simulink model "aerial_controller"  (R2026a)
settings: Solver=ode4  StopTime=2000  FixedStep=0.005
InitFcn:
  | addpath('C:\Users\banda\Documents\MATLAB\UAUV Control\Aerial');run('C:\Users\banda\Documents\MATLAB\UAUV Control\Aerial\aerial_init.m');run('C:\Users\banda\Documents\MATLAB\UAUV Control\Aerial\trajectory_aerial.m');update_trajectory_size('aerial_controller', size(trajectory,1));
values from neighbouring files (symbols this model uses):
  A_face = [0.1; 0.1; 0.2]    [aerial_init.m]    (also in underwater_init.m = [W_box * H_box)
  att_lim = 0.45    [aerial_init.m]
  Cd = [1.28; 1.28; 1.28]    [aerial_init.m]    (also in underwater_init.m = [1.2; 1.2; 1.5])
  g = 9.81    [aerial_init.m]    (also in underwater_init.m)
  i_lim_phi = 10.0    (= 10)    [aerial_init.m]
  i_lim_psi = 5.0    (= 5)    [aerial_init.m]
  i_lim_r = 5.0    (= 5)    [aerial_init.m]
  i_lim_t = 5.0    (= 5)    [aerial_init.m]
  i_lim_theta = 10.0    (= 10)    [aerial_init.m]
  i_lim_z = 10.0    (= 10)    [aerial_init.m]
  I_matrix = diag([Ixx, Iyy, Izz])    [aerial_init.m]
  Jr = 6.0e-5    (= 6e-05)    [aerial_init.m]
  Kd_phi = 18.39    [aerial_init.m]
  Kd_psi = 20.71    [aerial_init.m]
  Kd_r = 1.0    (= 1)    [aerial_init.m]
  Kd_t = 1.1    [aerial_init.m]
  Kd_theta = 45.6    [aerial_init.m]
  Kd_z = 2.0    (= 2)    [aerial_init.m]
  Ki_phi = 0.3    [aerial_init.m]
  Ki_psi = 0.1    [aerial_init.m]
  Ki_r = 0.02    [aerial_init.m]
  Ki_t = 0.02    [aerial_init.m]
  Ki_theta = 0.3    [aerial_init.m]
  Ki_z = 0.10    (= 0.1)    [aerial_init.m]
  Kp_phi = 61.4    [aerial_init.m]
  Kp_psi = 39.14    [aerial_init.m]
  Kp_r = 0.25    [aerial_init.m]
  Kp_t = 0.30    (= 0.3)    [aerial_init.m]
  Kp_theta = 198.1    [aerial_init.m]
  Kp_z = 1.00    (= 1)    [aerial_init.m]
  kQ = CQ_prop * rho_air * (D_prop^5) / (4 * pi^2)    (= 9.96442775246e-06)    [aerial_init.m]
  kT = CT_prop * rho_air * (D_prop^4) / (4 * pi^2)    (= 0.000495679441768)    [aerial_init.m]
  L_arm = 0.25    [aerial_init.m]
  m = 25.0    (= 25)    [aerial_init.m]    (also in underwater_init.m)
  r_tolerance = 2    [aerial_init.m]
  rho_air = 1.225    [aerial_init.m]
  tau_m = 0.06    [aerial_init.m]    (also in underwater_init.m)
  theta_tolerance = 0.4    [aerial_init.m]
  trajectory = [         6.00000000       0.00000000       0.00000000       0.00000000       0.00000000      -0.00100000       0.00000000       0.00000000      -0.28187976       3.14159265;         6.00000000       0.00000000      -2.06896552       0.00000000       0.00000000      -1.08000000       0.00000000       0.00000000      -0.09401790       3.14159265;         6.00000000       0.00000000      -4.13793103 ...(+46329 chars)    [trajectory_underwater.m]
  w_max = 700.0    (= 700)    [aerial_init.m]
  z_tolerance = 2    [aerial_init.m]
undefined symbols (not defined in the file or in its folder): DiscIntNeverNeededParam, x0
settings Model: Creator=banda  LastModifiedBy=banda

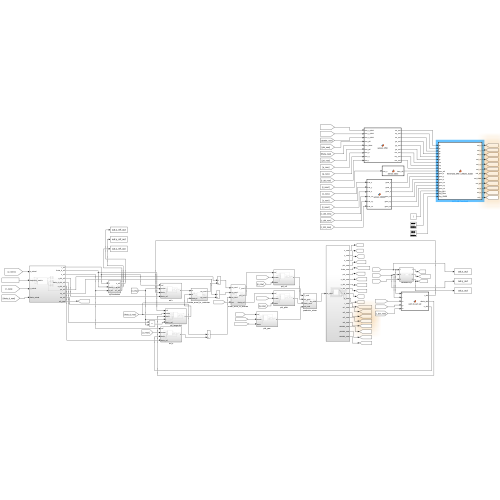
[thumbnail: Simulink's stored preview of the top-level diagram]
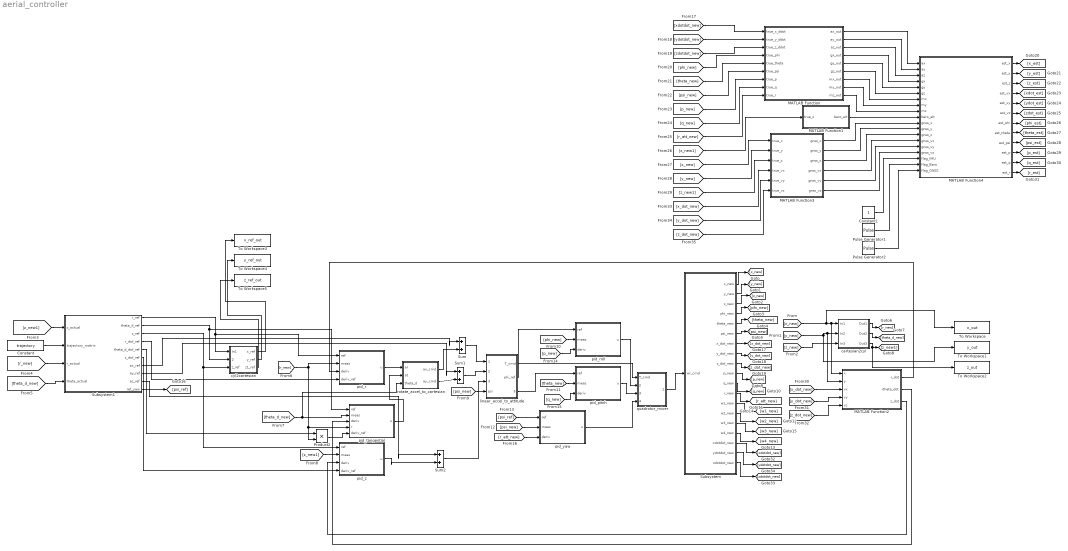
== system aerial_controller ==
  Constant : Constant  Value=trajectory
  Constant1 : Constant
  MATLAB Function : MATLAB Function  TreatAsAtomicUnit=on  SystemSampleTime=0.005
  MATLAB Function1 : MATLAB Function  TreatAsAtomicUnit=on  SystemSampleTime=0.02
  MATLAB Function2 : MATLAB Function  TreatAsAtomicUnit=on
  MATLAB Function3 : MATLAB Function  TreatAsAtomicUnit=on  SystemSampleTime=0.1
  MATLAB Function4 : MATLAB Function  TreatAsAtomicUnit=on  SystemSampleTime=0.005
  Product2 : Product
  Pulse Generator1 : DiscretePulseGenerator  Period=4  SampleTime=0.005
  Pulse Generator2 : DiscretePulseGenerator  Period=20  SampleTime=0.005
  Subsystem : Subsystem
  Subsystem1 : Subsystem  SystemSampleTime=0.05
  Sum : Sum  Inputs=|++
  Sum1 : Sum  Inputs=|++
  Sum2 : Sum  Inputs=|++
  To Workspace : ToWorkspace  VariableName=x_out  SaveFormat=Timeseries  SampleTime=-1
  To Workspace1 : ToWorkspace  VariableName=y_out  SaveFormat=Timeseries  SampleTime=-1
  To Workspace2 : ToWorkspace  VariableName=z_out  SaveFormat=Timeseries  SampleTime=-1
  To Workspace3 : ToWorkspace  VariableName=x_ref_out  SaveFormat=Timeseries  SampleTime=-1
  To Workspace4 : ToWorkspace  VariableName=y_ref_out  SaveFormat=Timeseries  SampleTime=-1
  To Workspace5 : ToWorkspace  VariableName=z_ref_out  SaveFormat=Timeseries  SampleTime=-1
  cartesian2cyl : Subsystem
  cyl2cartesian : Subsystem
  linear_accel_to_attitude : Subsystem
  pid_pitch : Subsystem
  pid_r : Subsystem
  pid_roll : Subsystem
  pid_tangential : Subsystem
  pid_yaw : Subsystem
  pid_z : Subsystem
  quadrotor_mixer : Subsystem
  rotate_accel_to_cartesian : Subsystem
  wires:
  Subsystem1/1(r_ref) -> cyl2cartesian/1(In1), pid_r/1(ref)
  Subsystem1/2(theta_d_ref) -> cyl2cartesian/2(theta_d_ref), pid_tangential/1(ref)
  Subsystem1/3(z_ref) -> pid_z/1(ref), cyl2cartesian/3(z_ref)
  MATLAB Function2/1(r_dot) -> pid_r/3(deriv)
  [x_new] -> To Workspace/1, MATLAB Function2/1(x), cartesian2cyl/1(In1)
  [y_new] -> MATLAB Function2/2(y), cartesian2cyl/2(In2), To Workspace1/1
  [z_new] -> cartesian2cyl/3(In3)
  cartesian2cyl/1(Out1) -> [r_new]
  cartesian2cyl/2(Out2) -> [theta_d_new]
  cartesian2cyl/3(Out3) -> To Workspace2/1, [z_new1]
  [r_new] -> Product2/2, pid_tangential/4(r), pid_r/2(meas)
  [theta_d_new] -> rotate_accel_to_cartesian/3(theta_d), pid_tangential/2(meas)
  [psi_new] -> linear_accel_to_attitude/4(psi)
  linear_accel_to_attitude/1(T_cmd) -> quadrotor_mixer/1(T_cmd)
  [psi_new] -> pid_yaw/2(meas)
  [r_att_new] -> pid_yaw/3(deriv)
  [x_dot_new] -> MATLAB Function2/3(vx)
  [y_dot_new] -> MATLAB Function2/4(vy)
  [z_dot_new] -> MATLAB Function2/5(vz)
  quadrotor_mixer/1(wr_cmd) -> Subsystem/1(wr_cmd)
  Subsystem/1(x_new) -> [x_new]
  Subsystem/4(phi_new) -> [phi_new]
  Subsystem/2(y_new) -> [y_new]
  Subsystem/5(theta_new) -> [theta_new]
  Subsystem/3(z_new) -> [z_new]
  Subsystem/6(psi_new) -> [psi_new]
  Subsystem/7(x_dot_new) -> [x_dot_new]
  Subsystem/8(y_dot_new) -> [y_dot_new]
  Subsystem/9(z_dot_new) -> [z_dot_new]
  Subsystem/10(p_new) -> [p_new]
  Subsystem/11(q_new) -> [q_new]
  Subsystem/12(r_new) -> [r_att_new]
  Subsystem/13(w1_new) -> [w1_new]
  Subsystem/14(w2_new) -> [w2_new]
  Subsystem/15(w3_new) -> [w3_new]
  Subsystem/16(w4_new) -> [w4_new]
  pid_r/1(u) -> rotate_accel_to_cartesian/1(ar)
  pid_tangential/1(u) -> rotate_accel_to_cartesian/2(at)
  pid_roll/1(u) -> quadrotor_mixer/2(phi_cmd)
  pid_pitch/1(u) -> quadrotor_mixer/3(theta_cmd)
  MATLAB Function2/2(rtheta_dot) -> pid_tangential/3(deriv)
  [z_new1] -> pid_z/2(meas)
  MATLAB Function2/3(z_dot) -> pid_z/3(deriv)
  linear_accel_to_attitude/2(phi_ref) -> pid_roll/1(ref)
  [phi_new] -> pid_roll/2(meas)
  [p_new] -> pid_roll/3(deriv)
  linear_accel_to_attitude/3(theta_ref) -> pid_pitch/1(ref)
  [theta_new] -> pid_pitch/2(meas)
  [q_new] -> pid_pitch/3(deriv)
  pid_yaw/1(u) -> quadrotor_mixer/4(psi_cmd)
  Subsystem1/5(theta_d_dot_ref) -> Product2/1
  Product2/1 -> pid_tangential/5(deriv_ref)
  Subsystem1/6(z_dot_ref) -> pid_z/4(deriv_ref)
  Subsystem1/4(r_dot_ref) -> pid_r/4(deriv_ref)
  rotate_accel_to_cartesian/1(ax_cmd) -> Sum/2
  Sum/1 -> linear_accel_to_attitude/1(ax_cmd)
  Subsystem1/7(ax_ref) -> Sum/1
  Sum1/1 -> linear_accel_to_attitude/2(ay_cmd)
  rotate_accel_to_cartesian/2(ay_cmd) -> Sum1/2
  Subsystem1/8(ay_ref) -> Sum1/1
  Sum2/1 -> linear_accel_to_attitude/3(az_cmd)
  Subsystem1/9(az_ref) -> Sum2/1
  Constant/1 -> Subsystem1/2(trajectory_matrix)
  [z_new1] -> Subsystem1/1(z_actual)
  Subsystem1/10(ref_yaw) -> [psi_ref]
  [psi_ref] -> pid_yaw/1(ref)
  cyl2cartesian/1(x_ref) -> To Workspace3/1
  cyl2cartesian/2(y_ref) -> To Workspace4/1
  cyl2cartesian/3(z1_ref) -> To Workspace5/1
  [r_new] -> Subsystem1/3(r_actual)
  [theta_d_new] -> Subsystem1/4(theta_actual)
  pid_z/1(u) -> Sum2/2
  MATLAB Function/1(ax_out) -> MATLAB Function4/1(ax)
  MATLAB Function/2(ay_out) -> MATLAB Function4/2(ay)
  MATLAB Function/3(az_out) -> MATLAB Function4/3(az)
  MATLAB Function/4(gx_out) -> MATLAB Function4/4(gx)
  MATLAB Function/5(gy_out) -> MATLAB Function4/5(gy)
  MATLAB Function/6(gz_out) -> MATLAB Function4/6(gz)
  MATLAB Function/7(mx_out) -> MATLAB Function4/7(mx)
  MATLAB Function/8(my_out) -> MATLAB Function4/8(my)
  MATLAB Function/9(mz_out) -> MATLAB Function4/9(mz)
  MATLAB Function1/1(baro_alt) -> MATLAB Function4/10(baro_alt)
  MATLAB Function3/1(gnss_x) -> MATLAB Function4/11(gnss_x)
  MATLAB Function3/2(gnss_y) -> MATLAB Function4/12(gnss_y)
  MATLAB Function3/3(gnss_z) -> MATLAB Function4/13(gnss_z)
  MATLAB Function3/4(gnss_vx) -> MATLAB Function4/14(gnss_vx)
  MATLAB Function3/5(gnss_vy) -> MATLAB Function4/15(gnss_vy)
  MATLAB Function3/6(gnss_vz) -> MATLAB Function4/16(gnss_vz)
  Constant1/1 -> MATLAB Function4/17(flag_IMU)
  Pulse Generator1/1 -> MATLAB Function4/18(flag_Baro)
  Pulse Generator2/1 -> MATLAB Function4/19(flag_GNSS)
  MATLAB Function4/2(est_y) -> [y_est]
  MATLAB Function4/1(est_x) -> [x_est]
  MATLAB Function4/12(est_r) -> [r_est]
  MATLAB Function4/11(est_q) -> [q_est]
  MATLAB Function4/10(est_p) -> [p_est]
  MATLAB Function4/9(est_psi) -> [psi_est]
  MATLAB Function4/8(est_theta) -> [theta_est]
  MATLAB Function4/7(est_phi) -> [phi_est]
  MATLAB Function4/6(est_vz) -> [zdot_est]
  MATLAB Function4/3(est_z) -> [z_est]
  MATLAB Function4/4(est_vx) -> [xdot_est]
  MATLAB Function4/5(est_vy) -> [ydot_est]
  Subsystem/17(xdotdot_new) -> [xdotdot_new]
  Subsystem/18(ydotdot_new) -> [ydotdot_new]
  Subsystem/19(zdotdot_new) -> [zdotdot_new]
  [xdotdot_new] -> MATLAB Function/1(true_x_ddot)
  [ydotdot_new] -> MATLAB Function/2(true_y_ddot)
  [zdotdot_new] -> MATLAB Function/3(true_z_ddot)
  [phi_new] -> MATLAB Function/4(true_phi)
  [theta_new] -> MATLAB Function/5(true_theta)
  [psi_new] -> MATLAB Function/6(true_psi)
  [p_new] -> MATLAB Function/7(true_p)
  [q_new] -> MATLAB Function/8(true_q)
  [r_att_new] -> MATLAB Function/9(true_r)
  [z_new1] -> MATLAB Function1/1(true_z)
  [x_dot_new] -> MATLAB Function3/4(true_vx)
  [y_dot_new] -> MATLAB Function3/5(true_vy)
  [z_dot_new] -> MATLAB Function3/6(true_vz)
  [x_new] -> MATLAB Function3/1(true_x)
  [y_new] -> MATLAB Function3/2(true_y)
  [z_new1] -> MATLAB Function3/3(true_z)

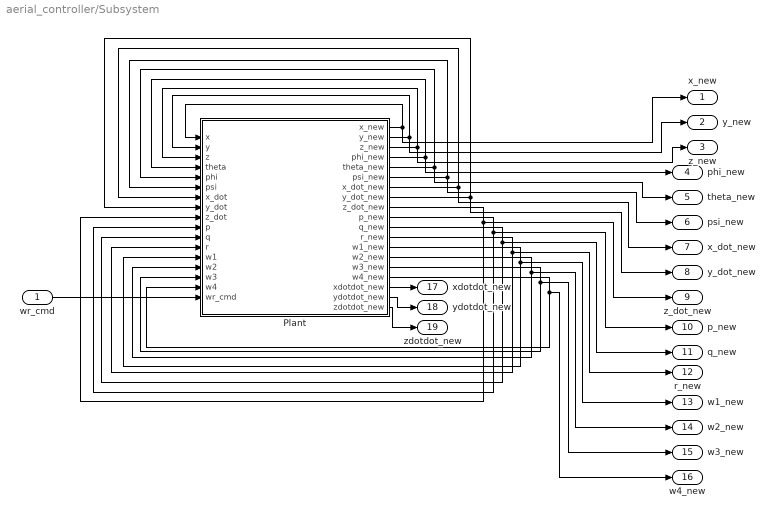
== system aerial_controller/Subsystem ==
  wr_cmd : Inport
  Plant : Subsystem
  x_new : Outport
  y_new : Outport  Port=2
  z_new : Outport  Port=3
  phi_new : Outport  Port=4
  theta_new : Outport  Port=5
  psi_new : Outport  Port=6
  x_dot_new : Outport  Port=7
  y_dot_new : Outport  Port=8
  z_dot_new : Outport  Port=9
  p_new : Outport  Port=10
  q_new : Outport  Port=11
  r_new : Outport  Port=12
  w1_new : Outport  Port=13
  w2_new : Outport  Port=14
  w3_new : Outport  Port=15
  w4_new : Outport  Port=16
  xdotdot_new : Outport  Port=17
  ydotdot_new : Outport  Port=18
  zdotdot_new : Outport  Port=19
  wires:
  Plant/3(z_new) -> z_new/1, Plant/3(z)
  Plant/2(y_new) -> y_new/1, Plant/2(y)
  Plant/9(z_dot_new) -> Plant/9(z_dot), z_dot_new/1
  Plant/8(y_dot_new) -> y_dot_new/1, Plant/8(y_dot)
  Plant/12(r_new) -> Plant/12(r), r_new/1
  Plant/1(x_new) -> x_new/1, Plant/1(x)
  Plant/5(theta_new) -> theta_new/1, Plant/5(phi)
  Plant/16(w4_new) -> Plant/16(w4), w4_new/1
  Plant/10(p_new) -> Plant/10(p), p_new/1
  wr_cmd/1 -> Plant/17(wr_cmd)
  Plant/11(q_new) -> Plant/11(q), q_new/1
  Plant/14(w2_new) -> Plant/14(w2), w2_new/1
  Plant/6(psi_new) -> psi_new/1, Plant/6(psi)
  Plant/7(x_dot_new) -> x_dot_new/1, Plant/7(x_dot)
  Plant/13(w1_new) -> Plant/13(w1), w1_new/1
  Plant/4(phi_new) -> phi_new/1, Plant/4(theta)
  Plant/15(w3_new) -> Plant/15(w3), w3_new/1
  Plant/17(xdotdot_new) -> xdotdot_new/1
  Plant/18(ydotdot_new) -> ydotdot_new/1
  Plant/19(zdotdot_new) -> zdotdot_new/1

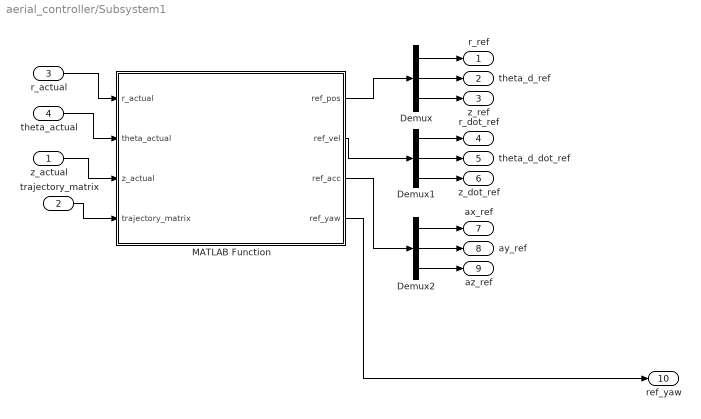
== system aerial_controller/Subsystem1 ==
  z_actual : Inport
  trajectory_matrix : Inport  Port=2
  r_actual : Inport  Port=3
  theta_actual : Inport  Port=4
  Demux : Demux  Outputs=3
  Demux1 : Demux  Outputs=3
  Demux2 : Demux  Outputs=3
  MATLAB Function : MATLAB Function  TreatAsAtomicUnit=on
  r_ref : Outport
  theta_d_ref : Outport  Port=2
  z_ref : Outport  Port=3
  r_dot_ref : Outport  Port=4
  theta_d_dot_ref : Outport  Port=5
  z_dot_ref : Outport  Port=6
  ax_ref : Outport  Port=7
  ay_ref : Outport  Port=8
  az_ref : Outport  Port=9
  ref_yaw : Outport  Port=10
  wires:
  Demux/2 -> theta_d_ref/1
  Demux1/2 -> theta_d_dot_ref/1
  Demux2/1 -> ax_ref/1
  MATLAB Function/2(ref_vel) -> Demux1/1
  Demux/1 -> r_ref/1
  MATLAB Function/3(ref_acc) -> Demux2/1
  Demux1/3 -> z_dot_ref/1
  Demux2/2 -> ay_ref/1
  Demux/3 -> z_ref/1
  trajectory_matrix/1 -> MATLAB Function/4(trajectory_matrix)
  Demux2/3 -> az_ref/1
  Demux1/1 -> r_dot_ref/1
  MATLAB Function/1(ref_pos) -> Demux/1
  z_actual/1 -> MATLAB Function/3(z_actual)
  MATLAB Function/4(ref_yaw) -> ref_yaw/1
  r_actual/1 -> MATLAB Function/1(r_actual)
  theta_actual/1 -> MATLAB Function/2(theta_actual)

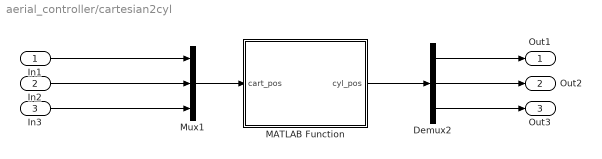
== system aerial_controller/cartesian2cyl ==
  In1 : Inport  PortDimensions=1
  In2 : Inport  Port=2  PortDimensions=1
  In3 : Inport  Port=3  PortDimensions=1
  Demux2 : Demux  Outputs=3
  MATLAB Function : MATLAB Function  TreatAsAtomicUnit=on
  Mux1 : Mux  Inputs=3
  Out1 : Outport  PortDimensions=1
  Out2 : Outport  Port=2  PortDimensions=1
  Out3 : Outport  Port=3  PortDimensions=1
  wires:
  Demux2/2 -> Out2/1
  In2/1 -> Mux1/2
  Mux1/1 -> MATLAB Function/1(cart_pos)
  In3/1 -> Mux1/3
  MATLAB Function/1(cyl_pos) -> Demux2/1
  Demux2/3 -> Out3/1
  Demux2/1 -> Out1/1
  In1/1 -> Mux1/1

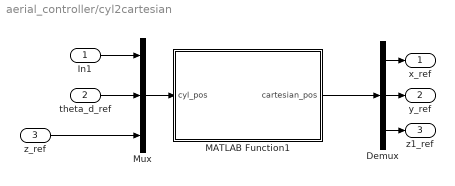
== system aerial_controller/cyl2cartesian ==
  In1 : Inport  PortDimensions=1
  theta_d_ref : Inport  Port=2  PortDimensions=1
  z_ref : Inport  Port=3  PortDimensions=1
  Demux : Demux  Outputs=3
  MATLAB Function1 : MATLAB Function  TreatAsAtomicUnit=on
  Mux : Mux  Inputs=3
  x_ref : Outport  PortDimensions=1
  y_ref : Outport  Port=2  PortDimensions=1
  z1_ref : Outport  Port=3  PortDimensions=1
  wires:
  theta_d_ref/1 -> Mux/2
  Mux/1 -> MATLAB Function1/1(cyl_pos)
  Demux/1 -> x_ref/1
  Demux/2 -> y_ref/1
  MATLAB Function1/1(cartesian_pos) -> Demux/1
  z_ref/1 -> Mux/3
  Demux/3 -> z1_ref/1
  In1/1 -> Mux/1

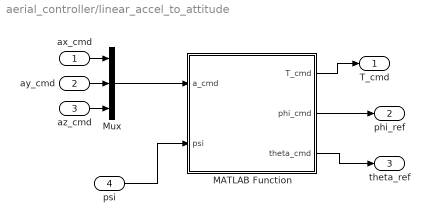
== system aerial_controller/linear_accel_to_attitude ==
  ax_cmd : Inport  PortDimensions=1
  ay_cmd : Inport  Port=2  PortDimensions=1
  az_cmd : Inport  Port=3  PortDimensions=1
  psi : Inport  Port=4  PortDimensions=1
  MATLAB Function : MATLAB Function  TreatAsAtomicUnit=on
  Mux : Mux  Inputs=3
  T_cmd : Outport  PortDimensions=1
  phi_ref : Outport  Port=2  PortDimensions=1
  theta_ref : Outport  Port=3  PortDimensions=1
  wires:
  psi/1 -> MATLAB Function/2(psi)
  Mux/1 -> MATLAB Function/1(a_cmd)
  ay_cmd/1 -> Mux/2
  ax_cmd/1 -> Mux/1
  az_cmd/1 -> Mux/3
  MATLAB Function/3(theta_cmd) -> theta_ref/1
  MATLAB Function/2(phi_cmd) -> phi_ref/1
  MATLAB Function/1(T_cmd) -> T_cmd/1

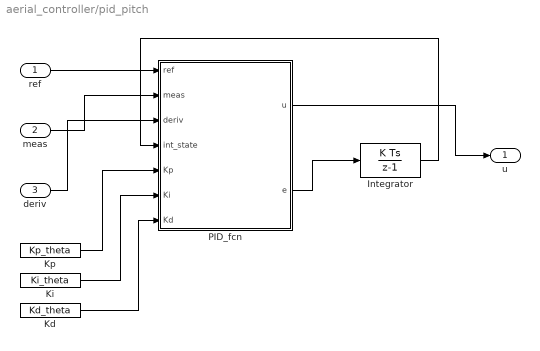
== system aerial_controller/pid_pitch ==
  ref : Inport
  meas : Inport  Port=2
  deriv : Inport  Port=3
  Integrator : DiscreteIntegrator  SampleTime=0.05  LimitOutput=on  UpperSaturationLimit=i_lim_theta  LowerSaturationLimit=-i_lim_theta  ICPrevOutput=DiscIntNeverNeededParam  ICPrevScaledInput=DiscIntNeverNeededParam
  Kd : Constant  Value=Kd_theta  OutDataTypeStr=double
  Ki : Constant  Value=Ki_theta  OutDataTypeStr=double
  Kp : Constant  Value=Kp_theta  OutDataTypeStr=double
  PID_fcn : MATLAB Function  TreatAsAtomicUnit=on
  u : Outport
  wires:
  ref/1 -> PID_fcn/1(ref)
  meas/1 -> PID_fcn/2(meas)
  deriv/1 -> PID_fcn/3(deriv)
  Integrator/1 -> PID_fcn/4(int_state)
  PID_fcn/1(u) -> u/1
  PID_fcn/2(e) -> Integrator/1
  Kp/1 -> PID_fcn/5(Kp)
  Ki/1 -> PID_fcn/6(Ki)
  Kd/1 -> PID_fcn/7(Kd)

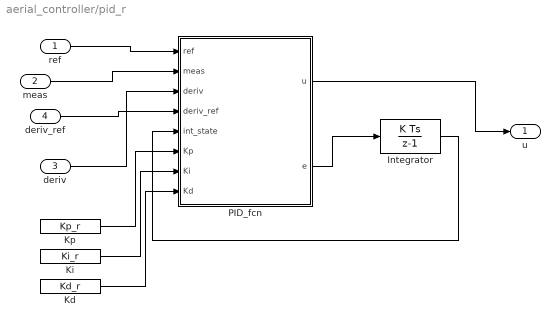
== system aerial_controller/pid_r ==
  ref : Inport
  meas : Inport  Port=2
  deriv : Inport  Port=3
  deriv_ref : Inport  Port=4
  Integrator : DiscreteIntegrator  SampleTime=0.05  LimitOutput=on  UpperSaturationLimit=i_lim_r  LowerSaturationLimit=-i_lim_r  ICPrevOutput=DiscIntNeverNeededParam  ICPrevScaledInput=DiscIntNeverNeededParam
  Kd : Constant  Value=Kd_r  OutDataTypeStr=double
  Ki : Constant  Value=Ki_r  OutDataTypeStr=double
  Kp : Constant  Value=Kp_r  OutDataTypeStr=double
  PID_fcn : MATLAB Function  TreatAsAtomicUnit=on
  u : Outport
  wires:
  ref/1 -> PID_fcn/1(ref)
  meas/1 -> PID_fcn/2(meas)
  deriv/1 -> PID_fcn/3(deriv)
  Integrator/1 -> PID_fcn/5(int_state)
  PID_fcn/1(u) -> u/1
  PID_fcn/2(e) -> Integrator/1
  Kp/1 -> PID_fcn/6(Kp)
  Ki/1 -> PID_fcn/7(Ki)
  Kd/1 -> PID_fcn/8(Kd)
  deriv_ref/1 -> PID_fcn/4(deriv_ref)

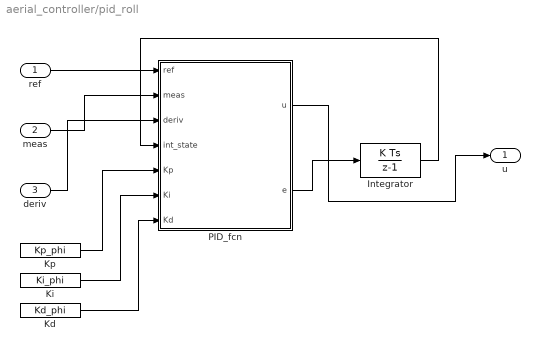
== system aerial_controller/pid_roll ==
  ref : Inport
  meas : Inport  Port=2
  deriv : Inport  Port=3
  Integrator : DiscreteIntegrator  SampleTime=0.05  LimitOutput=on  UpperSaturationLimit=i_lim_phi  LowerSaturationLimit=-i_lim_phi  ICPrevOutput=DiscIntNeverNeededParam  ICPrevScaledInput=DiscIntNeverNeededParam
  Kd : Constant  Value=Kd_phi  OutDataTypeStr=double
  Ki : Constant  Value=Ki_phi  OutDataTypeStr=double
  Kp : Constant  Value=Kp_phi  OutDataTypeStr=double
  PID_fcn : MATLAB Function  TreatAsAtomicUnit=on
  u : Outport
  wires:
  ref/1 -> PID_fcn/1(ref)
  meas/1 -> PID_fcn/2(meas)
  deriv/1 -> PID_fcn/3(deriv)
  Integrator/1 -> PID_fcn/4(int_state)
  PID_fcn/1(u) -> u/1
  PID_fcn/2(e) -> Integrator/1
  Kp/1 -> PID_fcn/5(Kp)
  Ki/1 -> PID_fcn/6(Ki)
  Kd/1 -> PID_fcn/7(Kd)

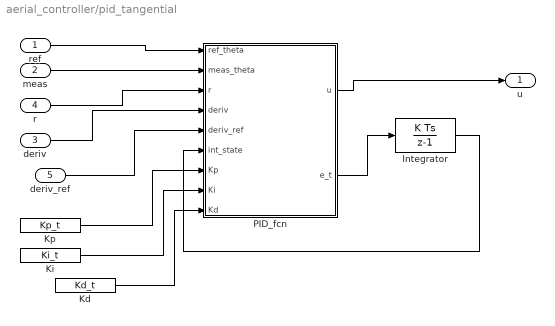
== system aerial_controller/pid_tangential ==
  ref : Inport
  meas : Inport  Port=2
  deriv : Inport  Port=3
  r : Inport  Port=4
  deriv_ref : Inport  Port=5
  Integrator : DiscreteIntegrator  SampleTime=0.05  LimitOutput=on  UpperSaturationLimit=i_lim_t  LowerSaturationLimit=-i_lim_t  ICPrevOutput=DiscIntNeverNeededParam  ICPrevScaledInput=DiscIntNeverNeededParam
  Kd : Constant  Value=Kd_t  OutDataTypeStr=double
  Ki : Constant  Value=Ki_t  OutDataTypeStr=double
  Kp : Constant  Value=Kp_t  OutDataTypeStr=double
  PID_fcn : MATLAB Function  TreatAsAtomicUnit=on
  u : Outport
  wires:
  ref/1 -> PID_fcn/1(ref_theta)
  meas/1 -> PID_fcn/2(meas_theta)
  deriv/1 -> PID_fcn/4(deriv)
  Integrator/1 -> PID_fcn/6(int_state)
  PID_fcn/1(u) -> u/1
  PID_fcn/2(e_t) -> Integrator/1
  Kp/1 -> PID_fcn/7(Kp)
  Ki/1 -> PID_fcn/8(Ki)
  Kd/1 -> PID_fcn/9(Kd)
  r/1 -> PID_fcn/3(r)
  deriv_ref/1 -> PID_fcn/5(deriv_ref)

== system aerial_controller/pid_yaw ==
  ref : Inport
  meas : Inport  Port=2
  deriv : Inport  Port=3
  Integrator : DiscreteIntegrator  SampleTime=0.05  LimitOutput=on  UpperSaturationLimit=i_lim_psi  LowerSaturationLimit=-i_lim_psi  ICPrevOutput=DiscIntNeverNeededParam  ICPrevScaledInput=DiscIntNeverNeededParam
  Kd : Constant  Value=Kd_psi  OutDataTypeStr=double
  Ki : Constant  Value=Ki_psi  OutDataTypeStr=double
  Kp : Constant  Value=Kp_psi  OutDataTypeStr=double
  PID_fcn : MATLAB Function  TreatAsAtomicUnit=on
  u : Outport
  wires:
  ref/1 -> PID_fcn/1(ref)
  meas/1 -> PID_fcn/2(meas)
  deriv/1 -> PID_fcn/3(deriv)
  Integrator/1 -> PID_fcn/4(int_state)
  PID_fcn/1(u) -> u/1
  PID_fcn/2(e) -> Integrator/1
  Kp/1 -> PID_fcn/5(Kp)
  Ki/1 -> PID_fcn/6(Ki)
  Kd/1 -> PID_fcn/7(Kd)

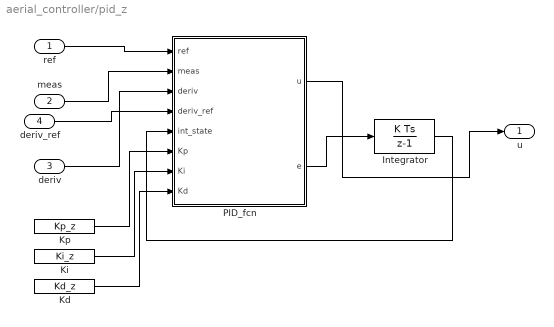
== system aerial_controller/pid_z ==
  ref : Inport
  meas : Inport  Port=2
  deriv : Inport  Port=3
  deriv_ref : Inport  Port=4
  Integrator : DiscreteIntegrator  SampleTime=0.05  LimitOutput=on  UpperSaturationLimit=i_lim_z  LowerSaturationLimit=-i_lim_z  ICPrevOutput=DiscIntNeverNeededParam  ICPrevScaledInput=DiscIntNeverNeededParam
  Kd : Constant  Value=Kd_z  OutDataTypeStr=double
  Ki : Constant  Value=Ki_z  OutDataTypeStr=double
  Kp : Constant  Value=Kp_z  OutDataTypeStr=double
  PID_fcn : MATLAB Function  TreatAsAtomicUnit=on
  u : Outport
  wires:
  ref/1 -> PID_fcn/1(ref)
  meas/1 -> PID_fcn/2(meas)
  deriv/1 -> PID_fcn/3(deriv)
  Integrator/1 -> PID_fcn/5(int_state)
  PID_fcn/1(u) -> u/1
  PID_fcn/2(e) -> Integrator/1
  Kp/1 -> PID_fcn/6(Kp)
  Ki/1 -> PID_fcn/7(Ki)
  Kd/1 -> PID_fcn/8(Kd)
  deriv_ref/1 -> PID_fcn/4(deriv_ref)

== system aerial_controller/quadrotor_mixer ==
  T_cmd : Inport  PortDimensions=1
  phi_cmd : Inport  Port=2  PortDimensions=1
  theta_cmd : Inport  Port=3  PortDimensions=1
  psi_cmd : Inport  Port=4  PortDimensions=1
  MATLAB Function : MATLAB Function  TreatAsAtomicUnit=on
  Mux : Mux
  wr_cmd : Outport  PortDimensions=4
  wires:
  Mux/1 -> MATLAB Function/1(u_virt)
  MATLAB Function/1(wr_cmd) -> wr_cmd/1
  psi_cmd/1 -> Mux/4
  phi_cmd/1 -> Mux/2
  theta_cmd/1 -> Mux/3
  T_cmd/1 -> Mux/1

== system aerial_controller/rotate_accel_to_cartesian ==
  ar : Inport  PortDimensions=1
  at : Inport  Port=2  PortDimensions=1
  theta_d : Inport  Port=3  PortDimensions=1
  Demux : Demux  Outputs=2
  MATLAB Function : MATLAB Function  TreatAsAtomicUnit=on
  Mux1 : Mux  Inputs=2
  ax_cmd : Outport  PortDimensions=1
  ay_cmd : Outport  Port=2  PortDimensions=1
  wires:
  Mux1/1 -> MATLAB Function/1(a_cyl)
  ar/1 -> Mux1/1
  MATLAB Function/1(a_cmd) -> Demux/1
  at/1 -> Mux1/2
  theta_d/1 -> MATLAB Function/2(theta_m)
  Demux/1 -> ax_cmd/1
  Demux/2 -> ay_cmd/1

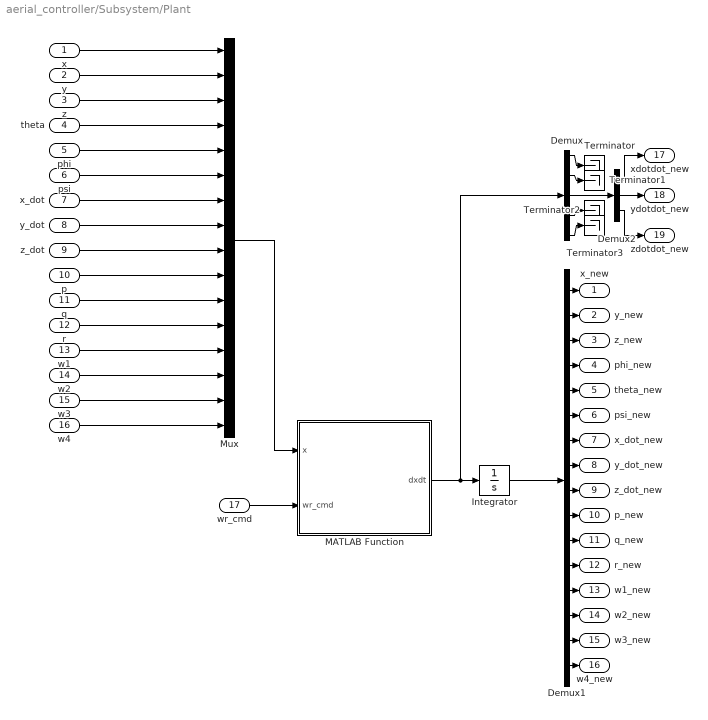
== system aerial_controller/Subsystem/Plant ==
  x : Inport
  y : Inport  Port=2
  z : Inport  Port=3
  theta : Inport  Port=4
  phi : Inport  Port=5
  psi : Inport  Port=6
  x_dot : Inport  Port=7
  y_dot : Inport  Port=8
  z_dot : Inport  Port=9
  p : Inport  Port=10
  q : Inport  Port=11
  r : Inport  Port=12
  w1 : Inport  Port=13
  w2 : Inport  Port=14
  w3 : Inport  Port=15
  w4 : Inport  Port=16
  wr_cmd : Inport  Port=17
  Demux : Demux  Outputs=5
  Demux1 : Demux  Outputs=16
  Demux2 : Demux  Outputs=3
  Integrator : Integrator  InitialCondition=x0
  MATLAB Function : MATLAB Function  TreatAsAtomicUnit=on
  Mux : Mux  Inputs=16
  Terminator{,1..3} (4 alike) : Terminator
  x_new : Outport  Tag=hello
  y_new : Outport  Port=2
  z_new : Outport  Port=3
  phi_new : Outport  Port=4
  theta_new : Outport  Port=5
  psi_new : Outport  Port=6
  x_dot_new : Outport  Port=7
  y_dot_new : Outport  Port=8
  z_dot_new : Outport  Port=9
  p_new : Outport  Port=10
  q_new : Outport  Port=11
  r_new : Outport  Port=12
  w1_new : Outport  Port=13
  w2_new : Outport  Port=14
  w3_new : Outport  Port=15
  w4_new : Outport  Port=16
  xdotdot_new : Outport  Port=17
  ydotdot_new : Outport  Port=18
  zdotdot_new : Outport  Port=19
  wires:
  MATLAB Function/1(dxdt) -> Demux/1, Integrator/1
  Integrator/1 -> Demux1/1
  Demux1/1 -> x_new/1
  Demux1/2 -> y_new/1
  Demux1/3 -> z_new/1
  Demux1/4 -> phi_new/1
  Demux1/5 -> theta_new/1
  Demux1/6 -> psi_new/1
  Demux1/7 -> x_dot_new/1
  Demux1/8 -> y_dot_new/1
  Demux1/9 -> z_dot_new/1
  Demux1/10 -> p_new/1
  Demux1/11 -> q_new/1
  Demux1/12 -> r_new/1
  Demux1/13 -> w1_new/1
  Demux1/14 -> w2_new/1
  Demux1/15 -> w3_new/1
  Demux1/16 -> w4_new/1
  x/1 -> Mux/1
  y/1 -> Mux/2
  z/1 -> Mux/3
  phi/1 -> Mux/5
  theta/1 -> Mux/4
  psi/1 -> Mux/6
  y_dot/1 -> Mux/8
  x_dot/1 -> Mux/7
  z_dot/1 -> Mux/9
  q/1 -> Mux/11
  p/1 -> Mux/10
  r/1 -> Mux/12
  w2/1 -> Mux/14
  w1/1 -> Mux/13
  w3/1 -> Mux/15
  w4/1 -> Mux/16
  wr_cmd/1 -> MATLAB Function/2(wr_cmd)
  Mux/1 -> MATLAB Function/1(x)
  Demux/3 -> Demux2/1
  Demux/1 -> Terminator/1
  Demux/2 -> Terminator1/1
  Demux/4 -> Terminator2/1
  Demux/5 -> Terminator3/1
  Demux2/1 -> xdotdot_new/1
  Demux2/2 -> ydotdot_new/1
  Demux2/3 -> zdotdot_new/1

== matlab function aerial_controller/quadrotor_mixer/MATLAB Function ==
  data: u_virt input; wr_cmd output; L_arm parameter; kT parameter; kQ parameter; w_max parameter
function wr_cmd = quadrotor_mixer(u_virt, L_arm, kT, kQ, w_max)
    wr_cmd = zeros(4,1);
    u_virt = reshape(u_virt, 4, 1);
    L_arm=L_arm(1); kT=kT(1); kQ=kQ(1); w_max=w_max(1);
    T_cmd=u_virt(1); tau_phi=u_virt(2); tau_theta=u_virt(3); tau_psi=u_virt(4);
    l_eff = (L_arm / sqrt(2)) * kT;
    A_mix = [ kT,     kT,     kT,     kT;
              l_eff, -l_eff,  l_eff, -l_eff;
             -l_eff, -l_eff,  l_eff,  l_eff;
              kQ,    -kQ,    -kQ,     kQ ];
    wr_sq_cmd = A_mix \ [T_cmd; tau_phi; tau_theta; tau_psi];
    wr_sq_cmd = max(wr_sq_cmd, 0.0);
    wr_cmd = min(sqrt(wr_sq_cmd), w_max);
end

== matlab function aerial_controller/MATLAB Function ==
  data: true_x_ddot input; ax_out output; true_y_ddot input; true_z_ddot input; ay_out output; az_out output; true_phi input; true_theta input; true_psi input; true_p input; true_q input; true_r input; gx_out output; gy_out output; gz_out output; mx_out output; my_out output; mz_out output
function [ax_out, ay_out, az_out, gx_out, gy_out, gz_out, mx_out, my_out, mz_out] = sensor_IMU(true_x_ddot, true_y_ddot, true_z_ddot, true_phi, true_theta, true_psi, true_p, true_q, true_r)
% Models a 9-DOF IMU taking scalar inputs from the continuous plant
    
    % Standard Deviations
    sigma_accel = 0.05;  % m/s^2
    sigma_gyro  = 0.002; % rad/s
    sigma_mag   = 0.01;  % Gauss

    % Repack internally
    true_pos_ddot = [true_x_ddot; true_y_ddot; true_z_ddot];
    true_wb       = [true_p; true_q; true_r];

    % Rotation Matrix: Inertial (ENU) to Body (FLU)
    R_T = [ cos(true_psi)*cos(true_theta),                                     sin(true_psi)*cos(true_theta),                                    -sin(true_theta);
            cos(true_psi)*sin(true_theta)*sin(true_phi) - sin(true_psi)*cos(true_phi),  sin(true_psi)*sin(true_theta)*sin(true_phi) + cos(true_psi)*cos(true_phi),  cos(true_theta)*sin(true_phi);
            cos(true_psi)*sin(true_theta)*cos(true_phi) + sin(true_psi)*sin(true_phi),  sin(true_psi)*sin(true_theta)*cos(true_phi) - cos(true_psi)*sin(true_phi),  cos(true_theta)*cos(true_phi) ];

    % Accelerometer
    g_inertial = [0; 0; -9.81]; 
    specific_force = true_pos_ddot - g_inertial; 
    accel_body = (R_T * specific_force) + sigma_accel * randn(3,1);

    % Gyroscope
    gyro_body = true_wb + sigma_gyro * randn(3,1);

    % Magnetometer
    mag_body = (R_T * [1; 0; 0]) + sigma_mag * randn(3,1);
    
    % Unpack for scalar outputs
    ax_out = accel_body(1); ay_out = accel_body(2); az_out = accel_body(3);
    gx_out = gyro_body(1);  gy_out = gyro_body(2);  gz_out = gyro_body(3);
    mx_out = mag_body(1);   my_out = mag_body(2);   mz_out = mag_body(3);
end

== matlab function aerial_controller/pid_yaw/PID_fcn ==
  data: ref input double size=1; u output double size=1; meas input double size=1; deriv input double size=1; int_state input double size=1; e output double size=1; Kp input double size=1; Ki input double size=1; Kd input double size=1
function [u, e] = PID_fcn(ref, meas, deriv, int_state, Kp, Ki, Kd)
    u = 0.0;  e = 0.0;
    ref=ref(1); meas=meas(1); deriv=deriv(1); int_state=int_state(1);
    Kp=Kp(1); Ki=Ki(1); Kd=Kd(1);
    e_raw = ref - meas;
    e = atan2(sin(e_raw), cos(e_raw));
    u = Kp*e + Ki*int_state - Kd*deriv;
end

== matlab function aerial_controller/pid_r/PID_fcn ==
  data: ref input double size=1; u output double size=1; meas input double size=1; deriv input double size=1; deriv_ref input double size=1; int_state input double size=1; e output double size=1; Kp input double size=1; Ki input double size=1; Kd input double size=1
function [u, e] = PID_fcn(ref, meas, deriv, deriv_ref, int_state, Kp, Ki, Kd)
    u = 0.0;  e = 0.0;
    ref=ref(1); meas=meas(1); deriv=deriv(1); deriv_ref=deriv_ref(1); int_state=int_state(1);
    Kp=Kp(1); Ki=Ki(1); Kd=Kd(1);
    e     = ref - meas;
    u     = Kp*e + Ki*int_state + Kd*(deriv_ref - deriv);
end

== matlab function aerial_controller/pid_tangential/PID_fcn ==
  data: ref_theta input double size=1; u output double size=1; meas_theta input double size=1; r input double size=1; deriv input double size=1; deriv_ref input double size=1; int_state input double size=1; e_t output double size=1; Kp input double size=1; Ki input double size=1; Kd input double size=1
function [u, e_t] = PID_fcn(ref_theta, meas_theta, r, deriv, deriv_ref, int_state, Kp, Ki, Kd)
    u = 0.0;  e_t = 0.0;
    ref_theta=ref_theta(1); meas_theta=meas_theta(1); r=r(1);
    deriv=deriv(1); deriv_ref=deriv_ref(1); int_state=int_state(1);
    Kp=Kp(1); Ki=Ki(1); Kd=Kd(1);
    e_raw = ref_theta - meas_theta;
    e_wrap = atan2(sin(e_raw), cos(e_raw));
    e_t   = e_wrap * r;
    u     = Kp*e_t + Ki*int_state + Kd*(deriv_ref - deriv);
end

== matlab function aerial_controller/pid_z/PID_fcn ==
  data: ref input double size=1; u output double size=1; meas input double size=1; deriv input double size=1; deriv_ref input double size=1; int_state input double size=1; e output double size=1; Kp input double size=1; Ki input double size=1; Kd input double size=1
function [u, e] = PID_fcn(ref, meas, deriv, deriv_ref, int_state, Kp, Ki, Kd)
    u = 0.0;  e = 0.0;
    ref=ref(1); meas=meas(1); deriv=deriv(1); deriv_ref=deriv_ref(1); int_state=int_state(1);
    Kp=Kp(1); Ki=Ki(1); Kd=Kd(1);
    e     = ref - meas;
    u     = Kp*e + Ki*int_state + Kd*(deriv_ref - deriv);
end

== matlab function aerial_controller/pid_roll/PID_fcn ==
  data: ref input double size=1; u output double size=1; meas input double size=1; deriv input double size=1; int_state input double size=1; e output double size=1; Kp input double size=1; Ki input double size=1; Kd input double size=1
function [u, e] = PID_fcn(ref, meas, deriv, int_state, Kp, Ki, Kd)
    u = 0.0;  e = 0.0;
    ref=ref(1); meas=meas(1); deriv=deriv(1); int_state=int_state(1);
    Kp=Kp(1); Ki=Ki(1); Kd=Kd(1);
    e = ref - meas;
    u = Kp*e + Ki*int_state - Kd*deriv;
end

== matlab function aerial_controller/pid_pitch/PID_fcn ==
  data: ref input double size=1; u output double size=1; meas input double size=1; deriv input double size=1; int_state input double size=1; e output double size=1; Kp input double size=1; Ki input double size=1; Kd input double size=1
function [u, e] = PID_fcn(ref, meas, deriv, int_state, Kp, Ki, Kd)
    u = 0.0;  e = 0.0;
    ref=ref(1); meas=meas(1); deriv=deriv(1); int_state=int_state(1);
    Kp=Kp(1); Ki=Ki(1); Kd=Kd(1);
    e = ref - meas;
    u = Kp*e + Ki*int_state - Kd*deriv;
end

== matlab function aerial_controller/Subsystem1/MATLAB Function ==
  settings: updateMethod=DISCRETE
  data: r_actual input; theta_actual input; z_actual input double size=1; ref_pos output double size=[3,1]; trajectory_matrix input double size=[30244, 10]; ref_vel output double size=[3,1]; ref_acc output double size=[3,1]; z_tolerance parameter double size=1; ref_yaw output double size=1; r_tolerance parameter; theta_tolerance parameter
function [ref_pos, ref_vel, ref_acc, ref_yaw] = waypoint_manager(r_actual, theta_actual, z_actual, trajectory_matrix, z_tolerance, r_tolerance, theta_tolerance)
    % trajectory_matrix: Nx10 [r, theta, z, vr, vtheta, vz, ax, ay, az, yaw]
    % positions: cylindrical, velocities: cylindrical, accelerations: Cartesian
    % Dense trajectory (one row per dt=0.05s step) -- event trigger fires every step
    
    ref_pos = zeros(3,1);
    ref_vel = zeros(3,1);
    ref_acc = zeros(3,1);
    ref_yaw = 0.0;
    
    persistent wp_idx;
    if isempty(wp_idx)
        wp_idx = int32(1);
    end
    
    % Ensure scalar actuals and tolerances
    z_actual    = z_actual(1);
    z_tolerance = z_tolerance(1);
    target_z    = trajectory_matrix(wp_idx, 3);
    error_z     = abs(target_z - z_actual);
    
    theta_actual    = theta_actual(1);
    theta_tolerance = theta_tolerance(1);
    target_theta    = trajectory_matrix(wp_idx, 2);
    
    % FIX: Calculate shortest angular difference to handle wrap-around (-pi to pi)
    raw_diff    = target_theta - theta_actual;
    error_theta = abs(atan2(sin(raw_diff), cos(raw_diff)));
    
    r_actual    = r_actual(1);
    r_tolerance = r_tolerance(1);
    target_r    = trajectory_matrix(wp_idx, 1);
    error_r     = abs(target_r - r_actual);
    
    % Tolerance check (If failed, wp_idx remains unchanged)
    if error_z < z_tolerance && error_theta < theta_tolerance && error_r < r_tolerance
        if wp_idx < int32(size(trajectory_matrix, 1))
            wp_idx = wp_idx + int32(1);
        end
    end
    
    % Output current reference (will be the same as last step if tolerance check failed)
    ref_pos = trajectory_matrix(wp_idx, 1:3)';
    ref_vel = trajectory_matrix(wp_idx, 4:6)';
    ref_acc = trajectory_matrix(wp_idx, 7:9)';
    ref_yaw = trajectory_matrix(wp_idx, 10);
end

== matlab function aerial_controller/MATLAB Function1 ==
  data: true_z input; baro_alt output
function baro_alt = sensor_Baro(true_z)
% Models a Barometric Altimeter
    sigma_baro = 0.5; % meters 
    baro_alt = true_z + sigma_baro * randn(1,1);
end

== matlab function aerial_controller/MATLAB Function3 ==
  data: true_x input; gnss_x output; true_y input; true_z input; true_vx input; true_vy input; true_vz input; gnss_y output; gnss_z output; gnss_vx output; gnss_vy output; gnss_vz output
function [gnss_x, gnss_y, gnss_z, gnss_vx, gnss_vy, gnss_vz] = sensor_GNSS(true_x, true_y, true_z, true_vx, true_vy, true_vz)
% Models a GNSS/GPS Receiver
    sigma_pos = 1.5; % meters
    sigma_vel = 0.1; % m/s
    
    gnss_x = true_x + sigma_pos * randn(1,1);
    gnss_y = true_y + sigma_pos * randn(1,1);
    gnss_z = true_z + sigma_pos * randn(1,1);
    
    gnss_vx = true_vx + sigma_vel * randn(1,1);
    gnss_vy = true_vy + sigma_vel * randn(1,1);
    gnss_vz = true_vz + sigma_vel * randn(1,1);
end

== matlab function aerial_controller/MATLAB Function4 ==
  data: ax input; est_x output; ay input; az input; gx input; gy input; gz input; mx input; my input; mz input; baro_alt input; gnss_x input; gnss_y input; gnss_z input; gnss_vx input; gnss_vy input; gnss_vz input; flag_IMU input; flag_Baro input; flag_GNSS input; est_y output; est_z output; est_vx output; est_vy output; est_vz output; est_phi output; est_theta output; est_psi output; est_p output; est_q output; est_r output
function [est_x, est_y, est_z, est_vx, est_vy, est_vz, est_phi, est_theta, est_psi, est_p, est_q, est_r] = Kinematic_EKF_12State_Scalar(ax, ay, az, gx, gy, gz, mx, my, mz, baro_alt, gnss_x, gnss_y, gnss_z, gnss_vx, gnss_vy, gnss_vz, flag_IMU, flag_Baro, flag_GNSS)
% 12-State Kinematic EKF with scalar Simulink routing
    
    persistent x_est P_cov initialized
    
    if isempty(initialized)
        x_est = zeros(12, 1);
        P_cov = eye(12) * 10; 
        initialized = true;
    end
    
    dt = 0.005; % Base sample time (200Hz)
    g  = 9.81;

    % Repack measurements internally for matrix math
    accel    = [ax; ay; az];
    gyro     = [gx; gy; gz];
    mag      = [mx; my; mz];
    gnss_pos = [gnss_x; gnss_y; gnss_z];
    gnss_vel = [gnss_vx; gnss_vy; gnss_vz];

    % Tuning Parameters
    sigma_pos_noise  = 0.01;
    sigma_a_noise    = 1.5;  
    sigma_w_noise    = 0.1;  
    sigma_rate_rw    = 50.0; 

    Q = diag([ones(1,3)*sigma_pos_noise, ones(1,3)*sigma_a_noise, ones(1,3)*sigma_w_noise, ones(1,3)*sigma_rate_rw]) * dt^2;

    % =====================================================================
    % 1. PREDICTION STEP
    % =====================================================================
    if flag_IMU
        p_pos = x_est(1:3);
        v     = x_est(4:6);
        phi   = x_est(7); theta = x_est(8); psi = x_est(9);
        p_rate = x_est(10); q_rate = x_est(11); r_rate = x_est(12); 
        
        R = [ cos(psi)*cos(theta),  cos(psi)*sin(theta)*sin(phi) - sin(psi)*cos(phi),  cos(psi)*sin(theta)*cos(phi) + sin(psi)*sin(phi);
              sin(psi)*cos(theta),  sin(psi)*sin(theta)*sin(phi) + cos(psi)*cos(phi),  sin(psi)*sin(theta)*cos(phi) - cos(psi)*sin(phi);
             -sin(theta),           cos(theta)*sin(phi),                               cos(theta)*cos(phi) ];
             
        p_dot = v;
        v_dot = R * accel + [0; 0; -g];
        
        phi_dot   = p_rate + q_rate*sin(phi)*tan(theta) + r_rate*cos(phi)*tan(theta);
        theta_dot = q_rate*cos(phi) - r_rate*sin(phi);
        psi_dot   = q_rate*sin(phi)/cos(theta) + r_rate*cos(phi)/cos(theta);
        
        x_est(1:3) = p_pos + p_dot * dt;
        x_est(4:6) = v + v_dot * dt;
        x_est(7)   = phi + phi_dot * dt;
        x_est(8)   = theta + theta_dot * dt;
        x_est(9)   = psi + psi_dot * dt;
        
        F = eye(12);
        F(1:3, 4:6) = eye(3) * dt; 
        
        dvx_dphi = ay*(sin(psi)*sin(phi) + cos(psi)*cos(phi)*sin(theta)) + az*(sin(psi)*cos(phi) - cos(psi)*sin(phi)*sin(theta));
        dvx_dth  = ax*(-cos(psi)*sin(theta)) + ay*(cos(psi)*sin(phi)*cos(theta)) + az*(cos(psi)*cos(phi)*cos(theta));
        dvx_dpsi = ax*(-sin(psi)*cos(theta)) + ay*(-sin(psi)*sin(phi)*sin(theta) - cos(psi)*cos(phi)) + az*(-sin(psi)*cos(phi)*sin(theta) + cos(psi)*sin(phi));
        dvy_dphi = ay*(-cos(psi)*sin(phi) + sin(psi)*cos(phi)*sin(theta)) + az*(-cos(psi)*cos(phi) - sin(psi)*sin(phi)*sin(theta));
        dvy_dth  = ax*(-sin(psi)*sin(theta)) + ay*(sin(psi)*sin(phi)*cos(theta)) + az*(sin(psi)*cos(phi)*cos(theta));
        dvy_dpsi = ax*(cos(psi)*cos(theta)) + ay*(cos(psi)*sin(phi)*sin(theta) - sin(psi)*cos(phi)) + az*(cos(psi)*cos(phi)*sin(theta) + sin(psi)*sin(phi));
        dvz_dphi = ay*(cos(theta)*cos(phi)) + az*(-cos(theta)*sin(phi));
        dvz_dth  = ax*(-cos(theta)) + ay*(-sin(theta)*sin(phi)) + az*(-sin(theta)*cos(phi));
        
        F(4:6, 7:9) = [dvx_dphi, dvx_dth, dvx_dpsi;
                       dvy_dphi, dvy_dth, 0;
                       dvz_dphi, dvz_dth, 0] * dt;
                       
        F(7, 10:12) = [1, sin(phi)*tan(theta), cos(phi)*tan(theta)] * dt;
        F(8, 10:12) = [0, cos(phi),           -sin(phi)] * dt;
        F(9, 10:12) = [0, sin(phi)/cos(theta), cos(phi)/cos(theta)] * dt;
                       
        P_cov = F * P_cov * F' + Q;
    end

    % =====================================================================
    % 2. CORRECTION STEPS
    % =====================================================================
    
    if flag_IMU
        H_gyro = [zeros(3, 9), eye(3)];
        R_gyro = diag([0.005^2, 0.005^2, 0.005^2]); 
        S = H_gyro * P_cov * H_gyro' + R_gyro;
        K = P_cov * H_gyro' / S;
        y_res = gyro - H_gyro * x_est;
        x_est = x_est + K * y_res;
        P_cov = (eye(12) - K * H_gyro) * P_cov;
    end

    if flag_GNSS
        H_gnss = [eye(6), zeros(6,6)]; 
        R_gnss = diag([1.5^2, 1.5^2, 1.5^2, 0.1^2, 0.1^2, 0.1^2]); 
        z_gnss = [gnss_pos; gnss_vel];
        S = H_gnss * P_cov * H_gnss' + R_gnss;
        K = P_cov * H_gnss' / S;
        y_res = z_gnss - H_gnss * x_est;
        x_est = x_est + K * y_res;
        P_cov = (eye(12) - K * H_gnss) * P_cov;
    end
    
    if flag_Baro
        H_baro = zeros(1,12); H_baro(1,3) = 1; 
        R_baro = 0.5^2; 
        S = H_baro * P_cov * H_baro' + R_baro;
        K = P_cov * H_baro' / S;
        y_res = baro_alt - x_est(3);
        x_est = x_est + K * y_res;
        P_cov = (eye(12) - K * H_baro) * P_cov;
    end

    if flag_Baro 
        meas_yaw = atan2(mag(2), mag(1));
        H_mag = zeros(1,12); H_mag(1,9) = 1; 
        R_mag = 0.1^2; 
        S = H_mag * P_cov * H_mag' + R_mag;
        K = P_cov * H_mag' / S;
        y_res = meas_yaw - x_est(9);
        y_res = atan2(sin(y_res), cos(y_res)); 
        x_est = x_est + K * y_res;
        P_cov = (eye(12) - K * H_mag) * P_cov;
    end

    % Unpack estimate vector to scalar outputs
    est_x = x_est(1);   est_y = x_est(2);   est_z = x_est(3);
    est_vx = x_est(4);  est_vy = x_est(5);  est_vz = x_est(6);
    est_phi = x_est(7); est_theta = x_est(8); est_psi = x_est(9);
    est_p = x_est(10);  est_q = x_est(11);  est_r = x_est(12);
end

== matlab function aerial_controller/cyl2cartesian/MATLAB Function1 ==
  data: cyl_pos input; cartesian_pos output
function cartesian_pos = cyl2cartesian(cyl_pos)
    cartesian_pos = zeros(3,1);
    cyl_pos = reshape(cyl_pos, 3, 1);
    r = cyl_pos(1); theta = cyl_pos(2); z = cyl_pos(3);
    cartesian_pos = [r*cos(theta); r*sin(theta); z];
end

== matlab function aerial_controller/Subsystem/Plant/MATLAB Function ==
  data: dxdt output double size=[16,1]; x input double size=[16,1]; wr_cmd input double size=[4,1]; m parameter double size=1; g parameter double size=1; I_matrix parameter double size=[3,3]; rho_air parameter double size=1; kT parameter double size=1; L_arm parameter double size=1; kQ parameter double size=1; tau_m parameter double size=1; Jr parameter double size=1; Cd parameter double size=[3,1]; A_face parameter double size=[3,1]
function dxdt = quad_dynamics(x, wr_cmd, m, g, I_matrix, rho_air, kT, L_arm, kQ, tau_m, Jr, Cd, A_face)
% A_mix @ [w1^2 w2^2 w3^2 w4^2] = [T, tau_phi, tau_theta, tau_psi]
% X config, arms at 45 deg, tower between FL(1) and FR(2):
%
%   FL(1)  FR(2)        CCW: 1, 4   CW: 2, 3
%     \   /
%      \ /
%      / \
%     /   \
%   RL(3)  RR(4)
% ---------------------------------------------------------------------
% 1. DERIVED PARAMETERS (From Workspace Data)
% ---------------------------------------------------------------------
% The variables m, g, rho_air, I_matrix, kT, kQ, L_arm, tau_m, Jr, Cd, 
% and A_face are loaded from the Base Workspace as Parameters.
inv_I = inv(I_matrix);

% Effective moment arm for X-configuration
lx = (L_arm / sqrt(2)) * kT; 

% Forward Mixing Matrix (X-config: 1=FL(CCW), 2=FR(CW), 3=RL(CW), 4=RR(CCW))
% Maps true squared rotor speeds to actual Body Forces and Torques
A_mix = [ kT,   kT,   kT,   kT;
          lx,  -lx,   lx,  -lx;   % tau_phi
         -lx,  -lx,   lx,   lx;   % tau_theta
          kQ,  -kQ,  -kQ,   kQ ]; % tau_psi

% ---------------------------------------------------------------------
% 2. UNPACK THE CURRENT STATE VECTOR (16 States)
% ---------------------------------------------------------------------
% COLUMN ENFORCERS: Force Simulink inputs into strict column vectors 
% to prevent matrix dimension mismatch errors during multiplication.
x      = reshape(x,      16, 1);
wr_cmd = reshape(wr_cmd,  4, 1);
Cd     = Cd(:);
A_face = A_face(:);

% x(1:3)   = [x; y; z]                 (Inertial Position)
% x(4:6)   = [phi; theta; psi]         (Euler Angles ZYX - Attitude)
% x(7:9)   = [xd; yd; zd]              (Inertial Velocity)
% x(10:12) = [p; q; r]                 (Body Angular Rates)
% x(13:16) = [w1; w2; w3; w4]          (Actual Rotor Speeds)

pos   = x(1:3);
euler = x(4:6);
vel   = x(7:9);
wb    = reshape(x(10:12), 3, 1);
wr    = reshape(x(13:16), 4, 1);

phi   = euler(1);
theta = euler(2);  % Attitude pitch
psi   = euler(3);

% ---------------------------------------------------------------------
% 3. CALCULATE FORCES & TORQUES (DYNAMICS)
% ---------------------------------------------------------------------
% Actuator efforts from true rotor speeds
u_actual = A_mix * (wr.^2);
T        = u_actual(1);
tau_body = u_actual(2:4);

% Gyroscopic torque from rotors
Omega_net = wr(1) - wr(2) - wr(3) + wr(4);
tau_gyro  = Jr * Omega_net * [-wb(2); wb(1); 0.0];

% ZYX Euler Rotation Matrix (Body to Inertial)
R = [ cos(psi)*cos(theta),  cos(psi)*sin(theta)*sin(phi) - sin(psi)*cos(phi),  cos(psi)*sin(theta)*cos(phi) + sin(psi)*sin(phi);
      sin(psi)*cos(theta),  sin(psi)*sin(theta)*sin(phi) + cos(psi)*cos(phi),  sin(psi)*sin(theta)*cos(phi) - cos(psi)*sin(phi);
     -sin(theta),           cos(theta)*sin(phi),                               cos(theta)*cos(phi) ];
 
% Translational Forces
F_thrust = R * [0; 0; T];
F_grav   = [0; 0; -m * g];

% CORRECTED Aerodynamic Drag
v_rel_inertial = vel; % Assuming zero wind
v_rel_body     = R' * v_rel_inertial; % Transform velocity to Body Frame (using R transpose)

% Calculate drag physically in the Body Frame
F_drag_body = -0.5 * rho_air * (Cd .* A_face) .* v_rel_body .* abs(v_rel_body);

% Transform the resulting Drag Force back to the Inertial Frame
F_drag_inertial = R * F_drag_body;

% Accelerations (Newton-Euler)
% All forces are now properly aligned in the Inertial Frame
pos_ddot = (F_thrust + F_grav + F_drag_inertial) / m;
wb_dot   = inv_I * (tau_body - tau_gyro - cross(wb, I_matrix * wb));

% ---------------------------------------------------------------------
% 4. CALCULATE KINEMATICS & MOTOR LAG
% ---------------------------------------------------------------------
% Body rates to Euler rates
euler_kin = [ 1,  sin(phi)*sin(theta)/cos(theta),  cos(phi)*sin(theta)/cos(theta);
              0,  cos(phi),                       -sin(phi);
              0,  sin(phi)/cos(theta),             cos(phi)/cos(theta) ];
euler_dot = euler_kin * wb;

% First-order motor dynamics
wr_dot = (wr_cmd - wr) / tau_m;

% ---------------------------------------------------------------------
% 5. PACK DERIVATIVES INTO OUTPUT VECTOR
% ---------------------------------------------------------------------
dxdt = [vel; euler_dot; pos_ddot; wb_dot; wr_dot];
end

== matlab function aerial_controller/cartesian2cyl/MATLAB Function ==
  data: cart_pos input; cyl_pos output
function cyl_pos = cartesian2cyl(cart_pos)
    cyl_pos = zeros(3,1);
    cart_pos = reshape(cart_pos, 3, 1);
    x = cart_pos(1); y = cart_pos(2); z = cart_pos(3);
    r = sqrt(x^2 + y^2);
    r = max(r, 1e-6);   % clamp to avoid division by zero (matches Python r_m)
    cyl_pos = [r; atan2(y, x); z];
end

== matlab function aerial_controller/MATLAB Function2 ==
  data: x input; r_dot output; y input; vx input; vy input; vz input; rtheta_dot output; z_dot output
function [r_dot, rtheta_dot, z_dot] = cart_to_cyl_vel(x, y, vx, vy, vz)
    % Converts Cartesian velocity to cylindrical velocity components
    % rtheta_dot = r * theta_dot (arc-length tangential velocity [m/s])
    % consistent with the arc-length tangential error used in pid_tangential
    r_dot = 0.0; rtheta_dot = 0.0; z_dot = 0.0;
    x=x(1); y=y(1); vx=vx(1); vy=vy(1); vz=vz(1);
    r      = max(sqrt(x^2 + y^2), 1e-6);
    theta  = atan2(y, x);
    r_dot      = vx*cos(theta) + vy*sin(theta);
    rtheta_dot = -vx*sin(theta) + vy*cos(theta);  % = r * theta_dot
    z_dot      = vz;
end

== matlab function aerial_controller/rotate_accel_to_cartesian/MATLAB Function ==
  data: a_cyl input; a_cmd output; theta_m input
function a_cmd = rotate_accel_to_cartesian(a_cyl, theta_m)
    a_cmd = zeros(2,1);
    a_cyl = reshape(a_cyl, 2, 1);
    theta_m = theta_m(1);
    ar = a_cyl(1); at = a_cyl(2);
    a_cmd = [ar*cos(theta_m) - at*sin(theta_m);
             ar*sin(theta_m) + at*cos(theta_m)];
end

== matlab function aerial_controller/linear_accel_to_attitude/MATLAB Function ==
  data: a_cmd input; T_cmd output; psi input; phi_cmd output; theta_cmd output; m parameter; g parameter; att_lim parameter
function [T_cmd, phi_cmd, theta_cmd] = linear_accel_to_attitude(a_cmd, psi, m, g, att_lim)
    % Pre-initialize outputs as scalars so Coder can resolve dimensions
    T_cmd     = 0.0;
    phi_cmd   = 0.0;
    theta_cmd = 0.0;

    % Force scalar inputs
    a_cmd   = reshape(a_cmd, 3, 1);
    psi     = psi(1);
    m       = m(1);
    g       = g(1);
    att_lim = att_lim(1);

    % 1. Unpack acceleration command
    ax_cmd = a_cmd(1);
    ay_cmd = a_cmd(2);
    az_cmd = a_cmd(3);

    % 2. Total Thrust Command
    T_cmd_raw = m * (az_cmd + g);
    T_cmd     = max(T_cmd_raw, 0.1 * m * g);

    % 3. Pitch and Roll commands
    theta_raw = (ax_cmd * cos(psi) + ay_cmd * sin(psi)) * m / T_cmd;
    phi_raw   = (ax_cmd * sin(psi) - ay_cmd * cos(psi)) * m / T_cmd;

    % 4. Apply tilt limits
    theta_cmd = max(min(theta_raw, att_lim), -att_lim);
    phi_cmd   = max(min(phi_raw,   att_lim), -att_lim);
end
